simulink model "model"  (R2014a)
settings: Solver=ode45  StartTime=0.0  StopTime=10.0  MaxStep=0.01  RelTol=1e-3
values from neighbouring files (symbols this model uses):
  k1 = 10    [skrypt.m]
  k2 = 6    [skrypt.m]
undefined symbols (not defined in the file or in its folder): k3
settings Model: Creator=L13-4  LastModifiedBy=L13-4

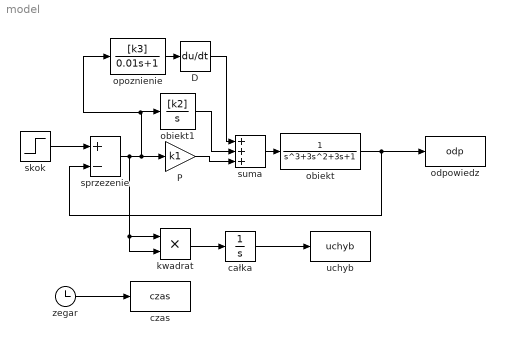
== system model ==
  D : Derivative
  P : Gain  Gain=k1
  całka : Integrator
  czas : ToWorkspace  VariableName=czas  SampleTime=-1
  kwadrat : Product
  obiekt : TransferFcn  Denominator=[1 3 3 1]
  obiekt1 : TransferFcn  Numerator=[k2]  Denominator=[1 0]
  odpowiedz : ToWorkspace  VariableName=odp  SampleTime=-1
  opoznienie : TransferFcn  Numerator=[k3]  Denominator=[0.01 1]
  skok : Step  SampleTime=0
  sprzezenie : Sum  Inputs=+-
  suma : Sum  Inputs=+++
  uchyb : ToWorkspace  VariableName=uchyb  SampleTime=-1
  zegar : Clock
  wires:
  skok/1 -> sprzezenie/1
  sprzezenie/1 -> obiekt1/1, opoznienie/1, P/1, kwadrat/1, kwadrat/2
  zegar/1 -> czas/1
  obiekt/1 -> odpowiedz/1, sprzezenie/2
  kwadrat/1 -> całka/1
  całka/1 -> uchyb/1
  suma/1 -> obiekt/1
  P/1 -> suma/3
  opoznienie/1 -> D/1
  D/1 -> suma/1
  obiekt1/1 -> suma/2
